simulink library "csu_ttl_time_to_level_lib"  (R2014b)
settings: Solver=ode45  StartTime=0.0  StopTime=10.0  RelTol=1e-3
undefined symbols (not defined in the file or in its folder): csc_cnt_dt, fsw_dt, sim_time_step_size
libraries: simulink x3
settings Model: Creator=Nilesh  LastModifiedBy=mstewart

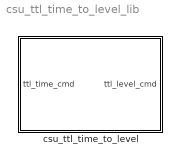
== system csu_ttl_time_to_level_lib ==
  csu_ttl_time_to_level : Subsystem

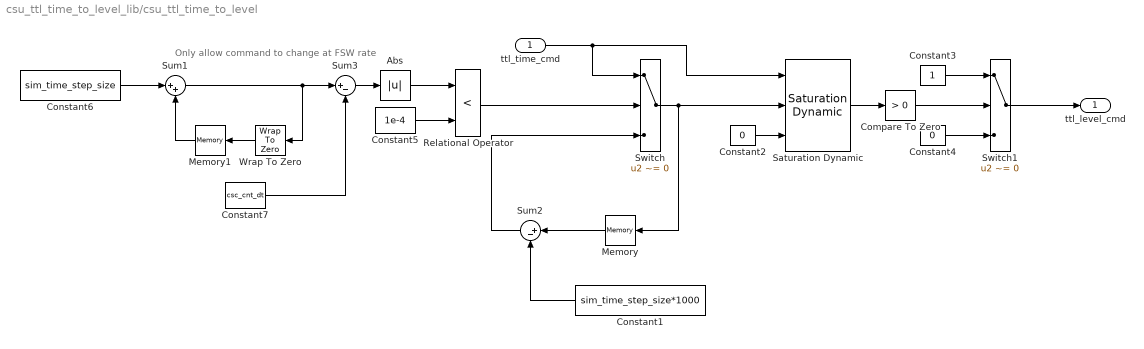
== system csu_ttl_time_to_level_lib/csu_ttl_time_to_level ==
  note: Only allow command to change at FSW rate
  ttl_time_cmd : Inport
  Abs : Abs
  Compare To Zero : simulink/Logic and Bit Operations/Compare To Zero  relop=>  OutDataTypeStr=boolean
  Constant1 : Constant  Value=sim_time_step_size*1000
  Constant2 : Constant  Value=0
  Constant3 : Constant  OutDataTypeStr=uint8
  Constant4 : Constant  Value=0  OutDataTypeStr=uint8
  Constant5 : Constant  Value=1e-4  OutDataTypeStr=double
  Constant6 : Constant  Value=sim_time_step_size  OutDataTypeStr=double
  Constant7 : Constant  Value=csc_cnt_dt  OutDataTypeStr=double
  Memory : Memory  InheritSampleTime=on
  Memory1 : Memory  X0=csc_cnt_dt - sim_time_step_size  InheritSampleTime=on
  Relational Operator : RelationalOperator  Operator=<  OutDataTypeStr=boolean
  Saturation Dynamic : simulink/Discontinuities/Saturation Dynamic  OutMin=[]  OutMax=[]  OutDataTypeStr=Inherit: Same as second input  OutDataType=fixdt(1, 16)  OutScaling=2^-10  DoSatur=off
  Sum1 : Sum  Inputs=|++
  Sum2 : Sum  Inputs=|+-
  Sum3 : Sum  Inputs=|+-
  Switch : Switch  Criteria=u2 ~= 0  Threshold=0.5
  Switch1 : Switch  Criteria=u2 ~= 0  Threshold=0.5
  Wrap To Zero : simulink/Discontinuities/Wrap To Zero  Threshold=fsw_dt*.99
  ttl_level_cmd : Outport
  wires:
  Constant5/1 -> Relational Operator/2
  Abs/1 -> Relational Operator/1
  Sum3/1 -> Abs/1
  Constant7/1 -> Sum3/2
  Constant6/1 -> Sum1/1
  Memory1/1 -> Sum1/2
  Wrap To Zero/1 -> Memory1/1
  Sum1/1 -> Sum3/1, Wrap To Zero/1
  ttl_time_cmd/1 -> Switch/1, Saturation Dynamic/1
  Constant1/1 -> Sum2/2
  Constant2/1 -> Saturation Dynamic/3
  Saturation Dynamic/1 -> Compare To Zero/1
  Constant3/1 -> Switch1/1
  Constant4/1 -> Switch1/3
  Sum2/1 -> Switch/3
  Switch1/1 -> ttl_level_cmd/1
  Relational Operator/1 -> Switch/2
  Compare To Zero/1 -> Switch1/2
  Switch/1 -> Memory/1, Saturation Dynamic/2
  Memory/1 -> Sum2/1
